simulink model "Electrical_System_2018b_obfs"  (R2019b)
settings: Solver=VariableStepAuto  StartTime=0.0  StopTime=5  RelTol=1e-3  AbsTol=1e-3  EnableMultiTasking=on
InitFcn:
  | Steady_State_Initialisation;
StopFcn:
  | %sscexplore(simlog);
  | %Logging
undefined symbols (not defined in the file): abrlhklxvp, aexgmhuedq, afmfmjnutg, afpphrjpnc, ahuxbyvruc, alarvljztt, amxnyqmnuw, aodrlwvqie, aolhmuplyq, aqpmguuqkg, auesgwirzl, aurophlnng, awamelrhru, ayfhvxflxn, azxkacuhqc, babszerikg, bawhdqanwq, bevoqecvei, bltjvqbchx, bmqsuewujl, bsmyqjfgnf, btvjbsmnve, bywgxqeadw, bziaduxaer, bzmcmdqocb, bzsvyvetat, ccsjnrbsih, cdvenygxwh, cedkrnslhx, cjheorclzs, cjrdshrtqx, ckhavyhcza, ckxewznhlz, cmrcgyiplk, conenicnws, cqkejbgjnn, csfnuwymhe, cunupkhwbh, cwzfvzuxxh, dcadmadufn, dcfponivnv, ddtrqjrhjn, dfhoxvkqas, dfrhtcwpne, dfvomcagjv, djijwylxea, dnmeqksrrm, dnzewbdkaa, dsqcykyxav, dtswwlttmm, ecumpidjtv, edegaywrct, ejjjsmnejc, eknqnehjdz, emvdetzouf, esxbqkbahr, etnkkbreiq, eunoiiiirw, ewewcuedir, fatkfxdhtc ... (+386)
libraries: fl_lib x802, ee_lib x362, fl_ps_legacy_lib x160, nesl_utility x85
(part 8 of 26)

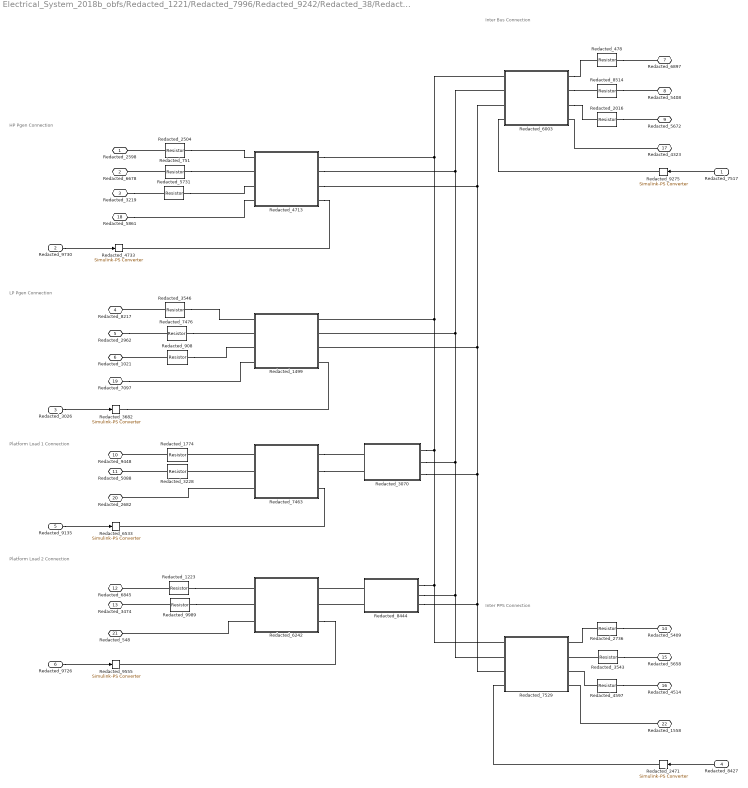
== system Electrical_System_2018b_obfs/Redacted_1221/Redacted_7996/Redacted_9242/Redacted_38/Redacted_8107 ==
  note: Inter Bus Connection
  note: Inter PPS Connection
  note: HP Pgen Connection
  note: LP Pgen Connection
  note: Platform Load 1 Connection
  note: Platform Load 2 Connection
  Redacted_7517 : Inport
  Redacted_9730 : Inport  Port=2
  Redacted_3026 : Inport  Port=3
  Redacted_8427 : Inport  Port=4
  Redacted_9135 : Inport  Port=5
  Redacted_9726 : Inport  Port=6
  Redacted_1223 : fl_lib/Electrical/Electrical Elements/Resistor  R=sjdolluzxe Ohm  i_specify=off  i_priority=None  i=ngzdomuwsd A  i_nominal_specify=off  i_nominal_unit=A  i_nominal_value=yvztmdkbhh  v_specify=off  v_priority=None  v=bscchvjlsd V  v_nominal_specify=off  v_nominal_unit=V  v_nominal_value=umzxrcvlku
  Redacted_1499 : Subsystem
      mask Display: image('SSPC.PNG'); % Use "Edit Image" on toolstrip to change.
  Redacted_1774 : fl_lib/Electrical/Electrical Elements/Resistor  R=ubcqenhdwv Ohm  i_specify=off  i_priority=None  i=lonqxilzul A  i_nominal_specify=off  i_nominal_unit=A  i_nominal_value=ngzkpdzjej  v_specify=off  v_priority=None  v=mtbfopdtqe V  v_nominal_specify=off  v_nominal_unit=V  v_nominal_value=ptvlyilmlu
  Redacted_2016 : fl_lib/Electrical/Electrical Elements/Resistor  R=uehuguxvnr Ohm  i_specify=off  i_priority=None  i=gpjoztugsb A  i_nominal_specify=off  i_nominal_unit=A  i_nominal_value=rxdsqmeito  v_specify=off  v_priority=None  v=mnwakbvrrh V  v_nominal_specify=off  v_nominal_unit=V  v_nominal_value=mnwzzbkphc
  Redacted_{2471,3682,4733,6533,9275,9555} (6 alike) : nesl_utility/Simulink-PS Converter  PhysicalDomain=network_engine_domain  SubClassName=ps_input  LeftPortType=input  RightPortType=output  PseudoPeriodic=off  Frequencies=[]  NoiseDistribution=none  NoiseParameters=[]  Unit=1  AffineConversion=off  FilteringAndDerivatives=provide  SimscapeFilterOrder=1  InputFilterTimeConstant=0.001  UdotUserProvided=0
  Redacted_2504 : fl_lib/Electrical/Electrical Elements/Resistor  R=awamelrhru Ohm  i_specify=off  i_priority=None  i=jnkfqgbyzv A  i_nominal_specify=off  i_nominal_unit=A  i_nominal_value=wkfpneyenj  v_specify=off  v_priority=None  v=rkhvctzjlt V  v_nominal_specify=off  v_nominal_unit=V  v_nominal_value=geiusuemea
  Redacted_2736 : fl_lib/Electrical/Electrical Elements/Resistor  R=ldsrjulotb Ohm  i_specify=off  i_priority=None  i=fblccdseua A  i_nominal_specify=off  i_nominal_unit=A  i_nominal_value=oeznhcqnka  v_specify=off  v_priority=None  v=npybdlghir V  v_nominal_specify=off  v_nominal_unit=V  v_nominal_value=gvfezcdtcn
  Redacted_3070 : Subsystem  VariantControlMode=Label  Variant=on  VariantControl=Variant1  LabelModeActiveChoice=Variant2
      mask Display: image('Rail Connection.png'); % Use "Edit Image" on toolstrip to change.
  Redacted_3228 : fl_lib/Electrical/Electrical Elements/Resistor  R=zdgwlscsrc Ohm  i_specify=off  i_priority=None  i=owjpacpnqo A  i_nominal_specify=off  i_nominal_unit=A  i_nominal_value=wwccxdknar  v_specify=off  v_priority=None  v=ackuqqmfxl V  v_nominal_specify=off  v_nominal_unit=V  v_nominal_value=wedppipphf
  Redacted_3543 : fl_lib/Electrical/Electrical Elements/Resistor  R=mrbtfyrlyp Ohm  i_specify=off  i_priority=None  i=kftbgibtup A  i_nominal_specify=off  i_nominal_unit=A  i_nominal_value=ldmyiogtiz  v_specify=off  v_priority=None  v=nnrgkdedip V  v_nominal_specify=off  v_nominal_unit=V  v_nominal_value=nkbhhfsxzn
  Redacted_3546 : fl_lib/Electrical/Electrical Elements/Resistor  R=jhgtovbypo Ohm  i_specify=off  i_priority=None  i=rlpegfrkjz A  i_nominal_specify=off  i_nominal_unit=A  i_nominal_value=oucwhhfkii  v_specify=off  v_priority=None  v=dysxsxinag V  v_nominal_specify=off  v_nominal_unit=V  v_nominal_value=uigskimzev
  Redacted_4597 : fl_lib/Electrical/Electrical Elements/Resistor  R=fvgznnouho Ohm  i_specify=off  i_priority=None  i=jphgmyadjd A  i_nominal_specify=off  i_nominal_unit=A  i_nominal_value=jndactudyu  v_specify=off  v_priority=None  v=lvpeuohgzz V  v_nominal_specify=off  v_nominal_unit=V  v_nominal_value=khxlxscugk
  Redacted_4713 : Subsystem
      mask Display: image('SSPC.PNG'); % Use "Edit Image" on toolstrip to change.
  Redacted_478 : fl_lib/Electrical/Electrical Elements/Resistor  R=hwfgewajfq Ohm  i_specify=off  i_priority=None  i=daiysladyz A  i_nominal_specify=off  i_nominal_unit=A  i_nominal_value=jmtrontctb  v_specify=off  v_priority=None  v=nojnagyxex V  v_nominal_specify=off  v_nominal_unit=V  v_nominal_value=ottkagceil
  Redacted_5731 : fl_lib/Electrical/Electrical Elements/Resistor  R=spitgjqwde Ohm  i_specify=off  i_priority=None  i=klwkvrfgdz A  i_nominal_specify=off  i_nominal_unit=A  i_nominal_value=waiewvjyul  v_specify=off  v_priority=None  v=itobauojdc V  v_nominal_specify=off  v_nominal_unit=V  v_nominal_value=nihyjnollp
  Redacted_6003 : Subsystem
      mask Display: image('SSPC.PNG'); % Use "Edit Image" on toolstrip to change.
  Redacted_6242 : Subsystem
      mask Display: image('SSPC.PNG'); % Use "Edit Image" on toolstrip to change.
  Redacted_7463 : Subsystem
      mask Display: image('SSPC.PNG'); % Use "Edit Image" on toolstrip to change.
  Redacted_7476 : fl_lib/Electrical/Electrical Elements/Resistor  R=gldcydwjeb Ohm  i_specify=off  i_priority=None  i=hjdgndgkrl A  i_nominal_specify=off  i_nominal_unit=A  i_nominal_value=eutsapefwf  v_specify=off  v_priority=None  v=resgdhqgwk V  v_nominal_specify=off  v_nominal_unit=V  v_nominal_value=uxmfwrhjba
  Redacted_751 : fl_lib/Electrical/Electrical Elements/Resistor  R=vvqvpmkxck Ohm  i_specify=off  i_priority=None  i=qbvnbydwpr A  i_nominal_specify=off  i_nominal_unit=A  i_nominal_value=fgrbwwnblb  v_specify=off  v_priority=None  v=wwcilqkvbu V  v_nominal_specify=off  v_nominal_unit=V  v_nominal_value=webjysbuft
  Redacted_7529 : Subsystem
      mask Display: image('SSPC.PNG'); % Use "Edit Image" on toolstrip to change.
  Redacted_8444 : Subsystem  VariantControlMode=Label  Variant=on  VariantControl=Variant1  LabelModeActiveChoice=Variant2
      mask Display: image('Rail Connection.png'); % Use "Edit Image" on toolstrip to change.
  Redacted_8514 : fl_lib/Electrical/Electrical Elements/Resistor  R=vfokesdqjr Ohm  i_specify=off  i_priority=None  i=owrhiolwzf A  i_nominal_specify=off  i_nominal_unit=A  i_nominal_value=lkozpfoafa  v_specify=off  v_priority=None  v=jqwzgqdxiv V  v_nominal_specify=off  v_nominal_unit=V  v_nominal_value=evvjvghatg
  Redacted_908 : fl_lib/Electrical/Electrical Elements/Resistor  R=bevoqecvei Ohm  i_specify=off  i_priority=None  i=jwlzzorzba A  i_nominal_specify=off  i_nominal_unit=A  i_nominal_value=rvqzfkktzi  v_specify=off  v_priority=None  v=bhosuphvek V  v_nominal_specify=off  v_nominal_unit=V  v_nominal_value=qozacnamyt
  Redacted_9989 : fl_lib/Electrical/Electrical Elements/Resistor  R=qrptpvdzui Ohm  i_specify=off  i_priority=None  i=aqwocztkwk A  i_nominal_specify=off  i_nominal_unit=A  i_nominal_value=pywwtpvidk  v_specify=off  v_priority=None  v=pgjzjpdwqq V  v_nominal_specify=off  v_nominal_unit=V  v_nominal_value=pfbusjnjhw
  Redacted_2598 : PMIOPort  Side=Left
  Redacted_6678 : PMIOPort  Port=2  Side=Left
  Redacted_3219 : PMIOPort  Port=3  Side=Left
  Redacted_8217 : PMIOPort  Port=4  Side=Left
  Redacted_2962 : PMIOPort  Port=5  Side=Left
  Redacted_1021 : PMIOPort  Port=6  Side=Left
  Redacted_6897 : PMIOPort  Port=7  Side=Right
  Redacted_5408 : PMIOPort  Port=8  Side=Right
  Redacted_5672 : PMIOPort  Port=9  Side=Right
  Redacted_9448 : PMIOPort  Port=10  Side=Left
  Redacted_5088 : PMIOPort  Port=11  Side=Left
  Redacted_6845 : PMIOPort  Port=12  Side=Left
  Redacted_3474 : PMIOPort  Port=13  Side=Left
  Redacted_5409 : PMIOPort  Port=14  Side=Right
  Redacted_5658 : PMIOPort  Port=15  Side=Right
  Redacted_4514 : PMIOPort  Port=16  Side=Right
  Redacted_4323 : PMIOPort  Port=17  Side=Left
  Redacted_5861 : PMIOPort  Port=18  Side=Left
  Redacted_7097 : PMIOPort  Port=19  Side=Left
  Redacted_2682 : PMIOPort  Port=20  Side=Left
  Redacted_548 : PMIOPort  Port=21  Side=Left
  Redacted_1558 : PMIOPort  Port=22  Side=Left
  wires:
  Redacted_9726/1 -> Redacted_9555/1
  Redacted_9135/1 -> Redacted_6533/1
  Redacted_8427/1 -> Redacted_2471/1
  Redacted_7517/1 -> Redacted_9275/1
  Redacted_3026/1 -> Redacted_3682/1
  Redacted_9730/1 -> Redacted_4733/1
  connections:
  Redacted_7463/RConn2 -- Redacted_3070/RConn2
  Redacted_7463/RConn1 -- Redacted_3070/RConn1
  Redacted_4713/RConn2 -- Redacted_7529/RConn2 -- Redacted_8444/LConn2 -- Redacted_3070/LConn2 -- Redacted_1499/RConn2 -- Redacted_6003/RConn2
  Redacted_4713/RConn1 -- Redacted_7529/RConn1 -- Redacted_8444/LConn1 -- Redacted_3070/LConn1 -- Redacted_1499/RConn1 -- Redacted_6003/RConn1
  Redacted_5731/LConn1 -- Redacted_4713/LConn3
  Redacted_751/RConn1 -- Redacted_6678/RConn1
  Redacted_908/LConn1 -- Redacted_1499/LConn3
  Redacted_7476/LConn1 -- Redacted_1499/LConn2
  Redacted_3546/LConn1 -- Redacted_1499/LConn1
  Redacted_7463/RConn3 -- Redacted_6533/RConn1
  Redacted_2471/RConn1 -- Redacted_7529/RConn4
  Redacted_6003/RConn4 -- Redacted_9275/RConn1
  Redacted_4713/RConn4 -- Redacted_4733/RConn1
  Redacted_3682/RConn1 -- Redacted_1499/RConn4
  Redacted_1774/RConn1 -- Redacted_9448/RConn1
  Redacted_2504/RConn1 -- Redacted_2598/RConn1
  Redacted_4713/RConn3 -- Redacted_7529/RConn3 -- Redacted_8444/LConn3 -- Redacted_3070/LConn3 -- Redacted_1499/RConn3 -- Redacted_6003/RConn3
  Redacted_9989/LConn1 -- Redacted_3474/RConn1
  Redacted_1223/RConn1 -- Redacted_6845/RConn1
  Redacted_3228/LConn1 -- Redacted_5088/RConn1
  Redacted_2504/LConn1 -- Redacted_4713/LConn1
  Redacted_751/LConn1 -- Redacted_4713/LConn2
  Redacted_3219/RConn1 -- Redacted_5731/RConn1
  Redacted_2736/LConn1 -- Redacted_7529/LConn1
  Redacted_3543/LConn1 -- Redacted_7529/LConn2
  Redacted_4597/LConn1 -- Redacted_7529/LConn3
  Redacted_4597/RConn1 -- Redacted_4514/RConn1
  Redacted_3543/RConn1 -- Redacted_5658/RConn1
  Redacted_2736/RConn1 -- Redacted_5409/RConn1
  Redacted_478/RConn1 -- Redacted_6897/RConn1
  Redacted_8514/RConn1 -- Redacted_5408/RConn1
  Redacted_2016/RConn1 -- Redacted_5672/RConn1
  Redacted_6003/LConn3 -- Redacted_2016/LConn1
  Redacted_6003/LConn2 -- Redacted_8514/LConn1
  Redacted_6003/LConn1 -- Redacted_478/LConn1
  Redacted_3546/RConn1 -- Redacted_8217/RConn1
  Redacted_2962/RConn1 -- Redacted_7476/RConn1
  Redacted_908/RConn1 -- Redacted_1021/RConn1
  Redacted_7463/LConn3 -- Redacted_2682/RConn1
  Redacted_1223/LConn1 -- Redacted_6242/LConn1
  Redacted_8444/RConn1 -- Redacted_6242/RConn1
  Redacted_9989/RConn1 -- Redacted_6242/LConn2
  Redacted_8444/RConn2 -- Redacted_6242/RConn2
  Redacted_6242/LConn3 -- Redacted_548/RConn1
  Redacted_6242/RConn3 -- Redacted_9555/RConn1
  Redacted_7463/LConn1 -- Redacted_1774/LConn1
  Redacted_7463/LConn2 -- Redacted_3228/RConn1
  Redacted_7097/RConn1 -- Redacted_1499/LConn4
  Redacted_5861/RConn1 -- Redacted_4713/LConn4
  Redacted_1558/RConn1 -- Redacted_7529/LConn4
  Redacted_4323/RConn1 -- Redacted_6003/LConn4

== system Electrical_System_2018b_obfs/Redacted_1221/Redacted_346/Redacted_5295/Redacted_9981/Redacted_313/Redacted_2425 ==
  Redacted_1003 : fl_lib/Electrical/Electrical Elements/Variable Resistor  Rmin=ucrhddlwym Ohm  i_specify=off  i_priority=None  i=lwddkcgiak A  i_nominal_specify=off  i_nominal_unit=A  i_nominal_value=dluejoekot  v_specify=off  v_priority=None  v=gabvqffkuy V  v_nominal_specify=off  v_nominal_unit=V  v_nominal_value=thskzrrjur
  Redacted_2194 : fl_lib/Electrical/Electrical Sensors/Voltage Sensor
  Redacted_7732 : fl_ps_legacy_lib/Legacy Physical Signals/Functions/PS Product
      settings: SourceProductName=Simscape  SourceProductBaseCode=SS
  Redacted_7738 : fl_lib/Physical Signals/Sources/PS Constant  constant=kcqbrxfpxd
  Redacted_9318 : fl_ps_legacy_lib/Legacy Physical Signals/Functions/PS Divide
      settings: SourceProductName=Simscape  SourceProductBaseCode=SS  InternalSimscapePortConfiguration="{\"Bottom\":[],\"Left\":[{\"id\":\"I1\",\"label\":\"\",\"type\":\"input\"},{\"id\":\"I2\",\"label\":\"\",\"type\":\"input\"}],\"Right\":[{\"id\":\"O\",\"label\":\"\",\"type\":\"output\"}],\"Top\":[]}"
  Redacted_7814 : PMIOPort  Side=Right
  Redacted_3087 : PMIOPort  Port=2  Side=Left
  connections:
  Redacted_2194/RConn2 -- Redacted_3087/RConn1 -- Redacted_1003/RConn1
  Redacted_7738/RConn1 -- Redacted_9318/LConn2
  Redacted_1003/LConn2 -- Redacted_7814/RConn1 -- Redacted_2194/LConn1
  Redacted_2194/RConn1 -- Redacted_7732/LConn1 -- Redacted_7732/LConn2
  Redacted_7732/RConn1 -- Redacted_9318/LConn1
  Redacted_1003/LConn1 -- Redacted_9318/RConn1

== system Electrical_System_2018b_obfs/Redacted_1221/Redacted_346/Redacted_5295/Redacted_9981/Redacted_313/Redacted_6908 ==
  Redacted_1859 : fl_ps_legacy_lib/Legacy Physical Signals/Functions/PS Divide
      settings: SourceProductName=Simscape  SourceProductBaseCode=SS  InternalSimscapePortConfiguration="{\"Bottom\":[],\"Left\":[{\"id\":\"I1\",\"label\":\"\",\"type\":\"input\"},{\"id\":\"I2\",\"label\":\"\",\"type\":\"input\"}],\"Right\":[{\"id\":\"O\",\"label\":\"\",\"type\":\"output\"}],\"Top\":[]}"
  Redacted_2395 : fl_lib/Physical Signals/Sources/PS Constant  constant=hefebkzejy
  Redacted_3767 : fl_ps_legacy_lib/Legacy Physical Signals/Functions/PS Product
      settings: SourceProductName=Simscape  SourceProductBaseCode=SS
  Redacted_6690 : fl_lib/Electrical/Electrical Sensors/Voltage Sensor
  Redacted_7700 : fl_ps_legacy_lib/Legacy Physical Signals/Functions/PS Divide
      settings: SourceProductName=Simscape  SourceProductBaseCode=SS  InternalSimscapePortConfiguration="{\"Bottom\":[],\"Left\":[{\"id\":\"I1\",\"label\":\"\",\"type\":\"input\"},{\"id\":\"I2\",\"label\":\"\",\"type\":\"input\"}],\"Right\":[{\"id\":\"O\",\"label\":\"\",\"type\":\"output\"}],\"Top\":[]}"
  Redacted_8220 : fl_lib/Electrical/Electrical Elements/Variable Resistor  Rmin=aoouqhrygj Ohm  i_specify=off  i_priority=None  i=ylcdblxypr A  i_nominal_specify=off  i_nominal_unit=A  i_nominal_value=tunconxvvm  v_specify=off  v_priority=None  v=slxuamdait V  v_nominal_specify=off  v_nominal_unit=V  v_nominal_value=jdedovsext
  Redacted_8956 : fl_lib/Electrical/Electrical Elements/Variable Resistor  Rmin=keflhiiijw Ohm  i_specify=off  i_priority=None  i=chkcspnvkh A  i_nominal_specify=off  i_nominal_unit=A  i_nominal_value=gilaklzvya  v_specify=off  v_priority=None  v=juwhcpfgoe V  v_nominal_specify=off  v_nominal_unit=V  v_nominal_value=srrbkqjtmp
  Redacted_8975 : fl_lib/Physical Signals/Sources/PS Constant  constant=otjyibokxj
  Redacted_4051 : PMIOPort  Side=Right
  Redacted_5582 : PMIOPort  Port=2  Side=Left
  connections:
  Redacted_6690/RConn2 -- Redacted_5582/RConn1 -- Redacted_8956/RConn1 -- Redacted_8220/RConn1
  Redacted_2395/RConn1 -- Redacted_1859/LConn2
  Redacted_8956/LConn1 -- Redacted_7700/RConn1
  Redacted_7700/LConn1 -- Redacted_1859/LConn1 -- Redacted_3767/RConn1
  Redacted_8220/LConn2 -- Redacted_4051/RConn1 -- Redacted_6690/LConn1 -- Redacted_8956/LConn2
  Redacted_8220/LConn1 -- Redacted_1859/RConn1
  Redacted_6690/RConn1 -- Redacted_3767/LConn1 -- Redacted_3767/LConn2
  Redacted_8975/RConn1 -- Redacted_7700/LConn2

== system Electrical_System_2018b_obfs/Redacted_1221/Redacted_346/Redacted_5295/Redacted_9981/Redacted_313/Redacted_7365 ==
  Redacted_2490 : fl_lib/Electrical/Electrical Elements/Variable Resistor  Rmin=aylmnucbgh Ohm  i_specify=off  i_priority=None  i=rgrzpfwzqo A  i_nominal_specify=off  i_nominal_unit=A  i_nominal_value=eloopaskyb  v_specify=off  v_priority=None  v=vsbpnvonuc V  v_nominal_specify=off  v_nominal_unit=V  v_nominal_value=kalqzgywlb
  Redacted_3163 : fl_lib/Electrical/Electrical Elements/Variable Resistor  Rmin=unppdegthn Ohm  i_specify=off  i_priority=None  i=jbvkybgull A  i_nominal_specify=off  i_nominal_unit=A  i_nominal_value=dgssyzjrzp  v_specify=off  v_priority=None  v=jamosoibqq V  v_nominal_specify=off  v_nominal_unit=V  v_nominal_value=lxrbzxzras
  Redacted_3458 : fl_lib/Physical Signals/Sources/PS Constant  constant=ubzmjljdyj
  Redacted_3580 : fl_lib/Electrical/Electrical Sensors/Voltage Sensor
  Redacted_5187 : fl_ps_legacy_lib/Legacy Physical Signals/Functions/PS Product
      settings: SourceProductName=Simscape  SourceProductBaseCode=SS
  Redacted_5260 : fl_ps_legacy_lib/Legacy Physical Signals/Functions/PS Divide
      settings: SourceProductName=Simscape  SourceProductBaseCode=SS  InternalSimscapePortConfiguration="{\"Bottom\":[],\"Left\":[{\"id\":\"I1\",\"label\":\"\",\"type\":\"input\"},{\"id\":\"I2\",\"label\":\"\",\"type\":\"input\"}],\"Right\":[{\"id\":\"O\",\"label\":\"\",\"type\":\"output\"}],\"Top\":[]}"
  Redacted_6111 : fl_ps_legacy_lib/Legacy Physical Signals/Functions/PS Divide
      settings: SourceProductName=Simscape  SourceProductBaseCode=SS  InternalSimscapePortConfiguration="{\"Bottom\":[],\"Left\":[{\"id\":\"I1\",\"label\":\"\",\"type\":\"input\"},{\"id\":\"I2\",\"label\":\"\",\"type\":\"input\"}],\"Right\":[{\"id\":\"O\",\"label\":\"\",\"type\":\"output\"}],\"Top\":[]}"
  Redacted_8313 : fl_lib/Physical Signals/Sources/PS Constant  constant=mhbishihtt
  Redacted_8633 : fl_lib/Physical Signals/Sources/PS Constant  constant=vqdfshvzpd
  Redacted_8641 : fl_lib/Electrical/Electrical Elements/Variable Resistor  Rmin=lceriuwihk Ohm  i_specify=off  i_priority=None  i=xhguggggch A  i_nominal_specify=off  i_nominal_unit=A  i_nominal_value=zwwgmbgpwt  v_specify=off  v_priority=None  v=jtqtzvsjjf V  v_nominal_specify=off  v_nominal_unit=V  v_nominal_value=koqitjzoac
  Redacted_8871 : fl_ps_legacy_lib/Legacy Physical Signals/Functions/PS Divide
      settings: SourceProductName=Simscape  SourceProductBaseCode=SS  InternalSimscapePortConfiguration="{\"Bottom\":[],\"Left\":[{\"id\":\"I1\",\"label\":\"\",\"type\":\"input\"},{\"id\":\"I2\",\"label\":\"\",\"type\":\"input\"}],\"Right\":[{\"id\":\"O\",\"label\":\"\",\"type\":\"output\"}],\"Top\":[]}"
  Redacted_4485 : PMIOPort  Side=Right
  Redacted_5454 : PMIOPort  Port=2  Side=Left
  connections:
  Redacted_8633/RConn1 -- Redacted_6111/LConn2
  Redacted_8871/LConn1 -- Redacted_6111/LConn1 -- Redacted_5260/LConn1 -- Redacted_5187/RConn1
  Redacted_3580/RConn1 -- Redacted_5187/LConn1 -- Redacted_5187/LConn2
  Redacted_3580/RConn2 -- Redacted_5454/RConn1 -- Redacted_2490/RConn1 -- Redacted_8641/RConn1 -- Redacted_3163/RConn1
  Redacted_8313/RConn1 -- Redacted_8871/LConn2
  Redacted_8641/LConn2 -- Redacted_3163/LConn2 -- Redacted_4485/RConn1 -- Redacted_3580/LConn1 -- Redacted_2490/LConn2
  Redacted_8641/LConn1 -- Redacted_8871/RConn1
  Redacted_3163/LConn1 -- Redacted_6111/RConn1
  Redacted_2490/LConn1 -- Redacted_5260/RConn1
  Redacted_3458/RConn1 -- Redacted_5260/LConn2

== system Electrical_System_2018b_obfs/Redacted_1221/Redacted_346/Redacted_6610/Redacted_2835/Redacted_9252/Redacted_1277 ==
  Redacted_2957 : fl_lib/Physical Signals/Sources/PS Constant  constant=hntxtbrvan
  Redacted_3289 : fl_ps_legacy_lib/Legacy Physical Signals/Functions/PS Divide
      settings: SourceProductName=Simscape  SourceProductBaseCode=SS  InternalSimscapePortConfiguration="{\"Bottom\":[],\"Left\":[{\"id\":\"I1\",\"label\":\"\",\"type\":\"input\"},{\"id\":\"I2\",\"label\":\"\",\"type\":\"input\"}],\"Right\":[{\"id\":\"O\",\"label\":\"\",\"type\":\"output\"}],\"Top\":[]}"
  Redacted_547 : fl_ps_legacy_lib/Legacy Physical Signals/Functions/PS Product
      settings: SourceProductName=Simscape  SourceProductBaseCode=SS
  Redacted_5585 : fl_ps_legacy_lib/Legacy Physical Signals/Functions/PS Divide
      settings: SourceProductName=Simscape  SourceProductBaseCode=SS  InternalSimscapePortConfiguration="{\"Bottom\":[],\"Left\":[{\"id\":\"I1\",\"label\":\"\",\"type\":\"input\"},{\"id\":\"I2\",\"label\":\"\",\"type\":\"input\"}],\"Right\":[{\"id\":\"O\",\"label\":\"\",\"type\":\"output\"}],\"Top\":[]}"
  Redacted_839 : fl_lib/Electrical/Electrical Elements/Variable Resistor  Rmin=ftusmicwfq Ohm  i_specify=off  i_priority=None  i=uklqcuznbi A  i_nominal_specify=off  i_nominal_unit=A  i_nominal_value=rddqoyatwv  v_specify=off  v_priority=None  v=tgjxgvnhur V  v_nominal_specify=off  v_nominal_unit=V  v_nominal_value=vnyslbtiig
  Redacted_8762 : fl_lib/Physical Signals/Sources/PS Constant  constant=jflishkqsg
  Redacted_9128 : fl_lib/Electrical/Electrical Elements/Variable Resistor  Rmin=qsdxrwkver Ohm  i_specify=off  i_priority=None  i=pdlhlzexxi A  i_nominal_specify=off  i_nominal_unit=A  i_nominal_value=yzkznragjx  v_specify=off  v_priority=None  v=qyfqyctmml V  v_nominal_specify=off  v_nominal_unit=V  v_nominal_value=bvyqzspggz
  Redacted_9715 : fl_lib/Electrical/Electrical Sensors/Voltage Sensor
  Redacted_724 : PMIOPort  Side=Right
  Redacted_3875 : PMIOPort  Port=2  Side=Left
  connections:
  Redacted_9715/RConn2 -- Redacted_3875/RConn1 -- Redacted_839/RConn1 -- Redacted_9128/RConn1
  Redacted_8762/RConn1 -- Redacted_5585/LConn2
  Redacted_839/LConn1 -- Redacted_3289/RConn1
  Redacted_3289/LConn1 -- Redacted_5585/LConn1 -- Redacted_547/RConn1
  Redacted_9128/LConn2 -- Redacted_724/RConn1 -- Redacted_9715/LConn1 -- Redacted_839/LConn2
  Redacted_9128/LConn1 -- Redacted_5585/RConn1
  Redacted_9715/RConn1 -- Redacted_547/LConn1 -- Redacted_547/LConn2
  Redacted_2957/RConn1 -- Redacted_3289/LConn2

== system Electrical_System_2018b_obfs/Redacted_1221/Redacted_346/Redacted_6610/Redacted_2835/Redacted_9252/Redacted_3806 ==
  Redacted_3118 : fl_ps_legacy_lib/Legacy Physical Signals/Functions/PS Product
      settings: SourceProductName=Simscape  SourceProductBaseCode=SS
  Redacted_3339 : fl_ps_legacy_lib/Legacy Physical Signals/Functions/PS Divide
      settings: SourceProductName=Simscape  SourceProductBaseCode=SS  InternalSimscapePortConfiguration="{\"Bottom\":[],\"Left\":[{\"id\":\"I1\",\"label\":\"\",\"type\":\"input\"},{\"id\":\"I2\",\"label\":\"\",\"type\":\"input\"}],\"Right\":[{\"id\":\"O\",\"label\":\"\",\"type\":\"output\"}],\"Top\":[]}"
  Redacted_3753 : fl_lib/Physical Signals/Sources/PS Constant  constant=bhqmgwpoeu
  Redacted_6387 : fl_lib/Electrical/Electrical Elements/Variable Resistor  Rmin=fsefuqbevk Ohm  i_specify=off  i_priority=None  i=wtglzyrwpk A  i_nominal_specify=off  i_nominal_unit=A  i_nominal_value=xsjlgnukht  v_specify=off  v_priority=None  v=hmnbvytqop V  v_nominal_specify=off  v_nominal_unit=V  v_nominal_value=kwwhelhhsh
  Redacted_6775 : fl_ps_legacy_lib/Legacy Physical Signals/Functions/PS Divide
      settings: SourceProductName=Simscape  SourceProductBaseCode=SS  InternalSimscapePortConfiguration="{\"Bottom\":[],\"Left\":[{\"id\":\"I1\",\"label\":\"\",\"type\":\"input\"},{\"id\":\"I2\",\"label\":\"\",\"type\":\"input\"}],\"Right\":[{\"id\":\"O\",\"label\":\"\",\"type\":\"output\"}],\"Top\":[]}"
  Redacted_7098 : fl_ps_legacy_lib/Legacy Physical Signals/Functions/PS Divide
      settings: SourceProductName=Simscape  SourceProductBaseCode=SS  InternalSimscapePortConfiguration="{\"Bottom\":[],\"Left\":[{\"id\":\"I1\",\"label\":\"\",\"type\":\"input\"},{\"id\":\"I2\",\"label\":\"\",\"type\":\"input\"}],\"Right\":[{\"id\":\"O\",\"label\":\"\",\"type\":\"output\"}],\"Top\":[]}"
  Redacted_7175 : fl_lib/Electrical/Electrical Sensors/Voltage Sensor
  Redacted_8063 : fl_lib/Electrical/Electrical Elements/Variable Resistor  Rmin=nkymtixsrf Ohm  i_specify=off  i_priority=None  i=ppisdarxxe A  i_nominal_specify=off  i_nominal_unit=A  i_nominal_value=ldesszfayy  v_specify=off  v_priority=None  v=otwcycsjqs V  v_nominal_specify=off  v_nominal_unit=V  v_nominal_value=yypjeaegtg
  Redacted_8840 : fl_lib/Electrical/Electrical Elements/Variable Resistor  Rmin=pzmcuzozvp Ohm  i_specify=off  i_priority=None  i=cwimwyhenp A  i_nominal_specify=off  i_nominal_unit=A  i_nominal_value=htxqjogdoz  v_specify=off  v_priority=None  v=xddpqbensy V  v_nominal_specify=off  v_nominal_unit=V  v_nominal_value=gkgmpwbztd
  Redacted_9021 : fl_lib/Physical Signals/Sources/PS Constant  constant=rmmelrcjew
  Redacted_9341 : fl_lib/Physical Signals/Sources/PS Constant  constant=ygdylemzaz
  Redacted_2522 : PMIOPort  Side=Right
  Redacted_8581 : PMIOPort  Port=2  Side=Left
  connections:
  Redacted_9021/RConn1 -- Redacted_3339/LConn2
  Redacted_6775/LConn1 -- Redacted_3339/LConn1 -- Redacted_7098/LConn1 -- Redacted_3118/RConn1
  Redacted_7175/RConn1 -- Redacted_3118/LConn1 -- Redacted_3118/LConn2
  Redacted_7175/RConn2 -- Redacted_8581/RConn1 -- Redacted_8840/RConn1 -- Redacted_8063/RConn1 -- Redacted_6387/RConn1
  Redacted_3753/RConn1 -- Redacted_6775/LConn2
  Redacted_8063/LConn2 -- Redacted_6387/LConn2 -- Redacted_2522/RConn1 -- Redacted_7175/LConn1 -- Redacted_8840/LConn2
  Redacted_8063/LConn1 -- Redacted_6775/RConn1
  Redacted_6387/LConn1 -- Redacted_3339/RConn1
  Redacted_8840/LConn1 -- Redacted_7098/RConn1
  Redacted_9341/RConn1 -- Redacted_7098/LConn2

== system Electrical_System_2018b_obfs/Redacted_1221/Redacted_346/Redacted_6610/Redacted_2835/Redacted_9252/Redacted_5568 ==
  Redacted_150 : fl_ps_legacy_lib/Legacy Physical Signals/Functions/PS Divide
      settings: SourceProductName=Simscape  SourceProductBaseCode=SS  InternalSimscapePortConfiguration="{\"Bottom\":[],\"Left\":[{\"id\":\"I1\",\"label\":\"\",\"type\":\"input\"},{\"id\":\"I2\",\"label\":\"\",\"type\":\"input\"}],\"Right\":[{\"id\":\"O\",\"label\":\"\",\"type\":\"output\"}],\"Top\":[]}"
  Redacted_8136 : fl_lib/Electrical/Electrical Elements/Variable Resistor  Rmin=kynlkgokkv Ohm  i_specify=off  i_priority=None  i=grooiuzwtk A  i_nominal_specify=off  i_nominal_unit=A  i_nominal_value=qqrguaowlq  v_specify=off  v_priority=None  v=zlcogmwcqt V  v_nominal_specify=off  v_nominal_unit=V  v_nominal_value=saetspikha
  Redacted_8154 : fl_ps_legacy_lib/Legacy Physical Signals/Functions/PS Product
      settings: SourceProductName=Simscape  SourceProductBaseCode=SS
  Redacted_8673 : fl_lib/Electrical/Electrical Sensors/Voltage Sensor
  Redacted_9172 : fl_lib/Physical Signals/Sources/PS Constant  constant=xqmylgdwta
  Redacted_6145 : PMIOPort  Side=Right
  Redacted_4538 : PMIOPort  Port=2  Side=Left
  connections:
  Redacted_8673/RConn2 -- Redacted_4538/RConn1 -- Redacted_8136/RConn1
  Redacted_9172/RConn1 -- Redacted_150/LConn2
  Redacted_8136/LConn2 -- Redacted_6145/RConn1 -- Redacted_8673/LConn1
  Redacted_8673/RConn1 -- Redacted_8154/LConn1 -- Redacted_8154/LConn2
  Redacted_8154/RConn1 -- Redacted_150/LConn1
  Redacted_8136/LConn1 -- Redacted_150/RConn1

== system Electrical_System_2018b_obfs/Redacted_1221/Redacted_7523/Redacted_5456/Redacted_1170/Redacted_7838/Redacted_5144 ==
  Redacted_1036 : fl_lib/Physical Signals/Sources/PS Constant  constant=jegtpryxoh
  Redacted_2543 : fl_ps_legacy_lib/Legacy Physical Signals/Functions/PS Divide
      settings: SourceProductName=Simscape  SourceProductBaseCode=SS  InternalSimscapePortConfiguration="{\"Bottom\":[],\"Left\":[{\"id\":\"I1\",\"label\":\"\",\"type\":\"input\"},{\"id\":\"I2\",\"label\":\"\",\"type\":\"input\"}],\"Right\":[{\"id\":\"O\",\"label\":\"\",\"type\":\"output\"}],\"Top\":[]}"
  Redacted_49 : fl_ps_legacy_lib/Legacy Physical Signals/Functions/PS Divide
      settings: SourceProductName=Simscape  SourceProductBaseCode=SS  InternalSimscapePortConfiguration="{\"Bottom\":[],\"Left\":[{\"id\":\"I1\",\"label\":\"\",\"type\":\"input\"},{\"id\":\"I2\",\"label\":\"\",\"type\":\"input\"}],\"Right\":[{\"id\":\"O\",\"label\":\"\",\"type\":\"output\"}],\"Top\":[]}"
  Redacted_5188 : fl_ps_legacy_lib/Legacy Physical Signals/Functions/PS Product
      settings: SourceProductName=Simscape  SourceProductBaseCode=SS
  Redacted_5777 : fl_lib/Physical Signals/Sources/PS Constant  constant=rcrmeoplpf
  Redacted_5890 : fl_lib/Electrical/Electrical Elements/Variable Resistor  Rmin=jbdockqooa Ohm  i_specify=off  i_priority=None  i=smzctytsfa A  i_nominal_specify=off  i_nominal_unit=A  i_nominal_value=sfdvwurekl  v_specify=off  v_priority=None  v=vkojlwtjgj V  v_nominal_specify=off  v_nominal_unit=V  v_nominal_value=xcctcsdmkc
  Redacted_916 : fl_lib/Electrical/Electrical Elements/Variable Resistor  Rmin=bduriqttnl Ohm  i_specify=off  i_priority=None  i=pzuombarcv A  i_nominal_specify=off  i_nominal_unit=A  i_nominal_value=iuerwcndbs  v_specify=off  v_priority=None  v=rlpmsqyvnw V  v_nominal_specify=off  v_nominal_unit=V  v_nominal_value=uebamzqyfb
  Redacted_9289 : fl_lib/Electrical/Electrical Elements/Variable Resistor  Rmin=fgxogjbchp Ohm  i_specify=off  i_priority=None  i=blrvskqthi A  i_nominal_specify=off  i_nominal_unit=A  i_nominal_value=vsmvaqbqsk  v_specify=off  v_priority=None  v=mgdzjmiklo V  v_nominal_specify=off  v_nominal_unit=V  v_nominal_value=guqxhtbrjs
  Redacted_9478 : fl_lib/Physical Signals/Sources/PS Constant  constant=stowntpskw
  Redacted_9535 : fl_lib/Electrical/Electrical Sensors/Voltage Sensor
  Redacted_9971 : fl_ps_legacy_lib/Legacy Physical Signals/Functions/PS Divide
      settings: SourceProductName=Simscape  SourceProductBaseCode=SS  InternalSimscapePortConfiguration="{\"Bottom\":[],\"Left\":[{\"id\":\"I1\",\"label\":\"\",\"type\":\"input\"},{\"id\":\"I2\",\"label\":\"\",\"type\":\"input\"}],\"Right\":[{\"id\":\"O\",\"label\":\"\",\"type\":\"output\"}],\"Top\":[]}"
  Redacted_2050 : PMIOPort  Side=Right
  Redacted_8541 : PMIOPort  Port=2  Side=Left
  connections:
  Redacted_1036/RConn1 -- Redacted_9971/LConn2
  Redacted_49/LConn1 -- Redacted_9971/LConn1 -- Redacted_2543/LConn1 -- Redacted_5188/RConn1
  Redacted_9535/RConn1 -- Redacted_5188/LConn1 -- Redacted_5188/LConn2
  Redacted_9535/RConn2 -- Redacted_8541/RConn1 -- Redacted_916/RConn1 -- Redacted_5890/RConn1 -- Redacted_9289/RConn1
  Redacted_5777/RConn1 -- Redacted_49/LConn2
  Redacted_5890/LConn2 -- Redacted_9289/LConn2 -- Redacted_2050/RConn1 -- Redacted_9535/LConn1 -- Redacted_916/LConn2
  Redacted_5890/LConn1 -- Redacted_49/RConn1
  Redacted_9289/LConn1 -- Redacted_9971/RConn1
  Redacted_916/LConn1 -- Redacted_2543/RConn1
  Redacted_9478/RConn1 -- Redacted_2543/LConn2

== system Electrical_System_2018b_obfs/Redacted_1221/Redacted_7523/Redacted_5456/Redacted_1170/Redacted_7838/Redacted_8977 ==
  Redacted_2057 : fl_ps_legacy_lib/Legacy Physical Signals/Functions/PS Divide
      settings: SourceProductName=Simscape  SourceProductBaseCode=SS  InternalSimscapePortConfiguration="{\"Bottom\":[],\"Left\":[{\"id\":\"I1\",\"label\":\"\",\"type\":\"input\"},{\"id\":\"I2\",\"label\":\"\",\"type\":\"input\"}],\"Right\":[{\"id\":\"O\",\"label\":\"\",\"type\":\"output\"}],\"Top\":[]}"
  Redacted_2371 : fl_ps_legacy_lib/Legacy Physical Signals/Functions/PS Product
      settings: SourceProductName=Simscape  SourceProductBaseCode=SS
  Redacted_4169 : fl_lib/Physical Signals/Sources/PS Constant  constant=miqgumozpq
  Redacted_4481 : fl_lib/Electrical/Electrical Elements/Variable Resistor  Rmin=awuncwxwbo Ohm  i_specify=off  i_priority=None  i=yzdjqdysyd A  i_nominal_specify=off  i_nominal_unit=A  i_nominal_value=hakbqanfgj  v_specify=off  v_priority=None  v=dzlvdjzicn V  v_nominal_specify=off  v_nominal_unit=V  v_nominal_value=wzhyfgnrut
  Redacted_8382 : fl_lib/Electrical/Electrical Sensors/Voltage Sensor
  Redacted_2028 : PMIOPort  Side=Right
  Redacted_5189 : PMIOPort  Port=2  Side=Left
  connections:
  Redacted_8382/RConn2 -- Redacted_5189/RConn1 -- Redacted_4481/RConn1
  Redacted_4169/RConn1 -- Redacted_2057/LConn2
  Redacted_4481/LConn2 -- Redacted_2028/RConn1 -- Redacted_8382/LConn1
  Redacted_8382/RConn1 -- Redacted_2371/LConn1 -- Redacted_2371/LConn2
  Redacted_2371/RConn1 -- Redacted_2057/LConn1
  Redacted_4481/LConn1 -- Redacted_2057/RConn1

== system Electrical_System_2018b_obfs/Redacted_1221/Redacted_7523/Redacted_5456/Redacted_1170/Redacted_7838/Redacted_9032 ==
  Redacted_3347 : fl_ps_legacy_lib/Legacy Physical Signals/Functions/PS Divide
      settings: SourceProductName=Simscape  SourceProductBaseCode=SS  InternalSimscapePortConfiguration="{\"Bottom\":[],\"Left\":[{\"id\":\"I1\",\"label\":\"\",\"type\":\"input\"},{\"id\":\"I2\",\"label\":\"\",\"type\":\"input\"}],\"Right\":[{\"id\":\"O\",\"label\":\"\",\"type\":\"output\"}],\"Top\":[]}"
  Redacted_3472 : fl_lib/Electrical/Electrical Sensors/Voltage Sensor
  Redacted_4648 : fl_lib/Electrical/Electrical Elements/Variable Resistor  Rmin=ilhagcepcy Ohm  i_specify=off  i_priority=None  i=txqkipenug A  i_nominal_specify=off  i_nominal_unit=A  i_nominal_value=lknsdsyyob  v_specify=off  v_priority=None  v=fprvwctgje V  v_nominal_specify=off  v_nominal_unit=V  v_nominal_value=ezydewgnex
  Redacted_6018 : fl_lib/Electrical/Electrical Elements/Variable Resistor  Rmin=tqeokogvsk Ohm  i_specify=off  i_priority=None  i=itlubfuvbg A  i_nominal_specify=off  i_nominal_unit=A  i_nominal_value=brcqbsoomb  v_specify=off  v_priority=None  v=dyrsfosulq V  v_nominal_specify=off  v_nominal_unit=V  v_nominal_value=fbptapolxk
  Redacted_6710 : fl_ps_legacy_lib/Legacy Physical Signals/Functions/PS Divide
      settings: SourceProductName=Simscape  SourceProductBaseCode=SS  InternalSimscapePortConfiguration="{\"Bottom\":[],\"Left\":[{\"id\":\"I1\",\"label\":\"\",\"type\":\"input\"},{\"id\":\"I2\",\"label\":\"\",\"type\":\"input\"}],\"Right\":[{\"id\":\"O\",\"label\":\"\",\"type\":\"output\"}],\"Top\":[]}"
  Redacted_6712 : fl_lib/Physical Signals/Sources/PS Constant  constant=rokxsqlbal
  Redacted_7218 : fl_lib/Physical Signals/Sources/PS Constant  constant=xtbcrtydyl
  Redacted_8404 : fl_ps_legacy_lib/Legacy Physical Signals/Functions/PS Product
      settings: SourceProductName=Simscape  SourceProductBaseCode=SS
  Redacted_4984 : PMIOPort  Side=Right
  Redacted_6998 : PMIOPort  Port=2  Side=Left
  connections:
  Redacted_3472/RConn2 -- Redacted_6998/RConn1 -- Redacted_4648/RConn1 -- Redacted_6018/RConn1
  Redacted_7218/RConn1 -- Redacted_3347/LConn2
  Redacted_4648/LConn1 -- Redacted_6710/RConn1
  Redacted_6710/LConn1 -- Redacted_3347/LConn1 -- Redacted_8404/RConn1
  Redacted_6018/LConn2 -- Redacted_4984/RConn1 -- Redacted_3472/LConn1 -- Redacted_4648/LConn2
  Redacted_6018/LConn1 -- Redacted_3347/RConn1
  Redacted_3472/RConn1 -- Redacted_8404/LConn1 -- Redacted_8404/LConn2
  Redacted_6712/RConn1 -- Redacted_6710/LConn2

== system Electrical_System_2018b_obfs/Redacted_1221/Redacted_7523/Redacted_5495/Redacted_794/Redacted_2986/Redacted_177 ==
  Redacted_1067 : fl_ps_legacy_lib/Legacy Physical Signals/Functions/PS Product
      settings: SourceProductName=Simscape  SourceProductBaseCode=SS
  Redacted_1500 : fl_ps_legacy_lib/Legacy Physical Signals/Functions/PS Divide
      settings: SourceProductName=Simscape  SourceProductBaseCode=SS  InternalSimscapePortConfiguration="{\"Bottom\":[],\"Left\":[{\"id\":\"I1\",\"label\":\"\",\"type\":\"input\"},{\"id\":\"I2\",\"label\":\"\",\"type\":\"input\"}],\"Right\":[{\"id\":\"O\",\"label\":\"\",\"type\":\"output\"}],\"Top\":[]}"
  Redacted_1730 : fl_ps_legacy_lib/Legacy Physical Signals/Functions/PS Divide
      settings: SourceProductName=Simscape  SourceProductBaseCode=SS  InternalSimscapePortConfiguration="{\"Bottom\":[],\"Left\":[{\"id\":\"I1\",\"label\":\"\",\"type\":\"input\"},{\"id\":\"I2\",\"label\":\"\",\"type\":\"input\"}],\"Right\":[{\"id\":\"O\",\"label\":\"\",\"type\":\"output\"}],\"Top\":[]}"
  Redacted_3177 : fl_lib/Electrical/Electrical Elements/Variable Resistor  Rmin=tlwspqlxdk Ohm  i_specify=off  i_priority=None  i=lhwzujexpl A  i_nominal_specify=off  i_nominal_unit=A  i_nominal_value=cmqjlldhje  v_specify=off  v_priority=None  v=inxzndqvek V  v_nominal_specify=off  v_nominal_unit=V  v_nominal_value=cspadccmef
  Redacted_4204 : fl_ps_legacy_lib/Legacy Physical Signals/Functions/PS Divide
      settings: SourceProductName=Simscape  SourceProductBaseCode=SS  InternalSimscapePortConfiguration="{\"Bottom\":[],\"Left\":[{\"id\":\"I1\",\"label\":\"\",\"type\":\"input\"},{\"id\":\"I2\",\"label\":\"\",\"type\":\"input\"}],\"Right\":[{\"id\":\"O\",\"label\":\"\",\"type\":\"output\"}],\"Top\":[]}"
  Redacted_4379 : fl_lib/Physical Signals/Sources/PS Constant  constant=mtjjkpbbtx
  Redacted_5113 : fl_lib/Physical Signals/Sources/PS Constant  constant=zheqgvokmf
  Redacted_6598 : fl_lib/Electrical/Electrical Elements/Variable Resistor  Rmin=oagjpbrwlb Ohm  i_specify=off  i_priority=None  i=iwhndvghwo A  i_nominal_specify=off  i_nominal_unit=A  i_nominal_value=xibvaeosbm  v_specify=off  v_priority=None  v=kbkjdnvnca V  v_nominal_specify=off  v_nominal_unit=V  v_nominal_value=cflqoyxhsq
  Redacted_6663 : fl_lib/Electrical/Electrical Elements/Variable Resistor  Rmin=hgdabcydmn Ohm  i_specify=off  i_priority=None  i=nlmbjlcaql A  i_nominal_specify=off  i_nominal_unit=A  i_nominal_value=zwsnkmlykp  v_specify=off  v_priority=None  v=bfjfgklnss V  v_nominal_specify=off  v_nominal_unit=V  v_nominal_value=nwnewssjzh
  Redacted_7070 : fl_lib/Electrical/Electrical Sensors/Voltage Sensor
  Redacted_8264 : fl_lib/Physical Signals/Sources/PS Constant  constant=lqbronwfpb
  Redacted_4029 : PMIOPort  Side=Right
  Redacted_6423 : PMIOPort  Port=2  Side=Left
  connections:
  Redacted_4379/RConn1 -- Redacted_1500/LConn2
  Redacted_1730/LConn1 -- Redacted_1500/LConn1 -- Redacted_4204/LConn1 -- Redacted_1067/RConn1
  Redacted_7070/RConn1 -- Redacted_1067/LConn1 -- Redacted_1067/LConn2
  Redacted_7070/RConn2 -- Redacted_6423/RConn1 -- Redacted_6598/RConn1 -- Redacted_3177/RConn1 -- Redacted_6663/RConn1
  Redacted_8264/RConn1 -- Redacted_1730/LConn2
  Redacted_3177/LConn2 -- Redacted_6663/LConn2 -- Redacted_4029/RConn1 -- Redacted_7070/LConn1 -- Redacted_6598/LConn2
  Redacted_3177/LConn1 -- Redacted_1730/RConn1
  Redacted_6663/LConn1 -- Redacted_1500/RConn1
  Redacted_6598/LConn1 -- Redacted_4204/RConn1
  Redacted_5113/RConn1 -- Redacted_4204/LConn2

== system Electrical_System_2018b_obfs/Redacted_1221/Redacted_7523/Redacted_5495/Redacted_794/Redacted_2986/Redacted_3587 ==
  Redacted_1494 : fl_ps_legacy_lib/Legacy Physical Signals/Functions/PS Product
      settings: SourceProductName=Simscape  SourceProductBaseCode=SS
  Redacted_223 : fl_lib/Electrical/Electrical Sensors/Voltage Sensor
  Redacted_3041 : fl_ps_legacy_lib/Legacy Physical Signals/Functions/PS Divide
      settings: SourceProductName=Simscape  SourceProductBaseCode=SS  InternalSimscapePortConfiguration="{\"Bottom\":[],\"Left\":[{\"id\":\"I1\",\"label\":\"\",\"type\":\"input\"},{\"id\":\"I2\",\"label\":\"\",\"type\":\"input\"}],\"Right\":[{\"id\":\"O\",\"label\":\"\",\"type\":\"output\"}],\"Top\":[]}"
  Redacted_6249 : fl_lib/Electrical/Electrical Elements/Variable Resistor  Rmin=uwqamwkwse Ohm  i_specify=off  i_priority=None  i=zksgjhowbn A  i_nominal_specify=off  i_nominal_unit=A  i_nominal_value=dkxnwexyzd  v_specify=off  v_priority=None  v=hxcmcrjjyr V  v_nominal_specify=off  v_nominal_unit=V  v_nominal_value=kwygmtklbv
  Redacted_8549 : fl_lib/Electrical/Electrical Elements/Variable Resistor  Rmin=opckuaijct Ohm  i_specify=off  i_priority=None  i=pesihwcwcy A  i_nominal_specify=off  i_nominal_unit=A  i_nominal_value=moicucijjn  v_specify=off  v_priority=None  v=bjcwcjmvax V  v_nominal_specify=off  v_nominal_unit=V  v_nominal_value=oqeosqjioe
  Redacted_8629 : fl_lib/Physical Signals/Sources/PS Constant  constant=uknecgagch
  Redacted_9447 : fl_ps_legacy_lib/Legacy Physical Signals/Functions/PS Divide
      settings: SourceProductName=Simscape  SourceProductBaseCode=SS  InternalSimscapePortConfiguration="{\"Bottom\":[],\"Left\":[{\"id\":\"I1\",\"label\":\"\",\"type\":\"input\"},{\"id\":\"I2\",\"label\":\"\",\"type\":\"input\"}],\"Right\":[{\"id\":\"O\",\"label\":\"\",\"type\":\"output\"}],\"Top\":[]}"
  Redacted_9605 : fl_lib/Physical Signals/Sources/PS Constant  constant=oseeykkvcq
  Redacted_2176 : PMIOPort  Side=Right
  Redacted_3086 : PMIOPort  Port=2  Side=Left
  connections:
  Redacted_223/RConn2 -- Redacted_3086/RConn1 -- Redacted_6249/RConn1 -- Redacted_8549/RConn1
  Redacted_8629/RConn1 -- Redacted_9447/LConn2
  Redacted_6249/LConn1 -- Redacted_3041/RConn1
  Redacted_3041/LConn1 -- Redacted_9447/LConn1 -- Redacted_1494/RConn1
  Redacted_8549/LConn2 -- Redacted_2176/RConn1 -- Redacted_223/LConn1 -- Redacted_6249/LConn2
  Redacted_8549/LConn1 -- Redacted_9447/RConn1
  Redacted_223/RConn1 -- Redacted_1494/LConn1 -- Redacted_1494/LConn2
  Redacted_9605/RConn1 -- Redacted_3041/LConn2

== system Electrical_System_2018b_obfs/Redacted_1221/Redacted_7523/Redacted_5495/Redacted_794/Redacted_2986/Redacted_9599 ==
  Redacted_114 : fl_ps_legacy_lib/Legacy Physical Signals/Functions/PS Divide
      settings: SourceProductName=Simscape  SourceProductBaseCode=SS  InternalSimscapePortConfiguration="{\"Bottom\":[],\"Left\":[{\"id\":\"I1\",\"label\":\"\",\"type\":\"input\"},{\"id\":\"I2\",\"label\":\"\",\"type\":\"input\"}],\"Right\":[{\"id\":\"O\",\"label\":\"\",\"type\":\"output\"}],\"Top\":[]}"
  Redacted_1426 : fl_ps_legacy_lib/Legacy Physical Signals/Functions/PS Product
      settings: SourceProductName=Simscape  SourceProductBaseCode=SS
  Redacted_2877 : fl_lib/Electrical/Electrical Elements/Variable Resistor  Rmin=wmhhprfely Ohm  i_specify=off  i_priority=None  i=rlsupiyusp A  i_nominal_specify=off  i_nominal_unit=A  i_nominal_value=cfqigqvwbc  v_specify=off  v_priority=None  v=tlikybqabe V  v_nominal_specify=off  v_nominal_unit=V  v_nominal_value=zjvecmhwwg
  Redacted_8928 : fl_lib/Physical Signals/Sources/PS Constant  constant=cquhzzrphq
  Redacted_9230 : fl_lib/Electrical/Electrical Sensors/Voltage Sensor
  Redacted_2019 : PMIOPort  Side=Right
  Redacted_8905 : PMIOPort  Port=2  Side=Left
  connections:
  Redacted_9230/RConn2 -- Redacted_8905/RConn1 -- Redacted_2877/RConn1
  Redacted_8928/RConn1 -- Redacted_114/LConn2
  Redacted_2877/LConn2 -- Redacted_2019/RConn1 -- Redacted_9230/LConn1
  Redacted_9230/RConn1 -- Redacted_1426/LConn1 -- Redacted_1426/LConn2
  Redacted_1426/RConn1 -- Redacted_114/LConn1
  Redacted_2877/LConn1 -- Redacted_114/RConn1
